simulink model "System_Function_Realization"  (R2019b)
settings: Solver=FixedStepAuto  StartTime=0.0  StopTime=10.0  FixedStep=0.2  RelTol=1e-3
model workspace (MAT data in the model file):
  a0 = 2
  a1 = -1
  b0 = 1
settings Model: Creator=Shreyas  LastModifiedBy=Shreyas
settings DataIOCC: SaveOutput=off  SaveTime=off

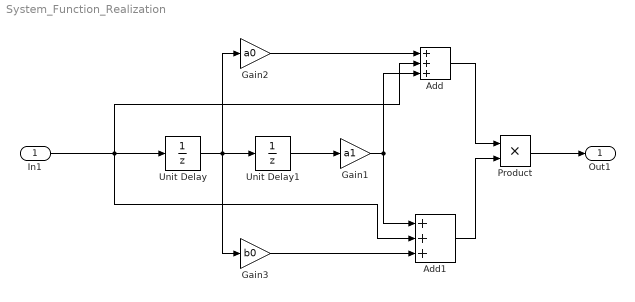
== system System_Function_Realization ==
  In1 : Inport  OutDataTypeStr=double  PortDimensions=1  SampleTime=[0.20000000000000001,0]
  Add : Sum  Inputs=+++
  Add1 : Sum  Inputs=+++
  Gain1 : Gain  Gain=a1
  Gain2 : Gain  Gain=a0
  Gain3 : Gain  Gain=b0
  Product : Product
  Unit Delay : UnitDelay  SampleTime=-1  HasFrameUpgradeWarning=on
  Unit Delay1 : UnitDelay  SampleTime=-1  HasFrameUpgradeWarning=on
  Out1 : Outport  OutDataTypeStr=double  PortDimensions=1  SampleTime=[0.20000000000000001,0]
  wires:
  Gain1/1 -> Add1/1, Add/3
  Product/1 -> Out1/1
  Add1/1 -> Product/2
  In1/1 -> Add/2, Unit Delay/1, Add1/2
  Gain2/1 -> Add/1
  Unit Delay/1 -> Gain3/1, Gain2/1, Unit Delay1/1
  Unit Delay1/1 -> Gain1/1
  Gain3/1 -> Add1/3
  Add/1 -> Product/1
